simulink model "bh_velocity_estimator"  (R2021a)
settings: Solver=ode15s  StartTime=0.0  StopTime=20  RelTol=1e-3
settings Model: Creator=bhorton  LastModifiedBy=bhorton

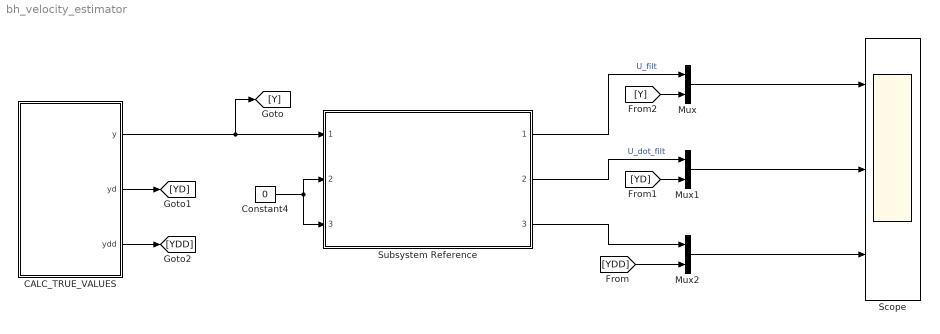
== system bh_velocity_estimator ==
  CALC_TRUE_VALUES : Subsystem
  Constant4 : Constant  Value=0
  Mux : Mux  Inputs=2
  Mux1 : Mux  Inputs=2
  Mux2 : Mux  Inputs=2
  Scope : Scope  NumInputPorts=3
  Subsystem Reference : Subsystem  ReferencedSubsystem=bh_COMPONENT_deriv_est  wn=2*pi*5000  p=1
  wires:
  CALC_TRUE_VALUES/1(y) -> [Y], Subsystem Reference/1
  Constant4/1 -> Subsystem Reference/3, Subsystem Reference/2
  Mux/1 -> Scope/1
  Mux1/1 -> Scope/2
  Mux2/1 -> Scope/3
  Subsystem Reference/1 -> Mux/1  "U_filt"
  Subsystem Reference/2 -> Mux1/1  "U_dot_filt"
  Subsystem Reference/3 -> Mux2/1
  CALC_TRUE_VALUES/3(ydd) -> [YDD]
  CALC_TRUE_VALUES/2(yd) -> [YD]
  [YDD] -> Mux2/2
  [YD] -> Mux1/2
  [Y] -> Mux/2

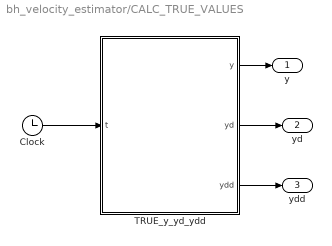
== system bh_velocity_estimator/CALC_TRUE_VALUES ==
  Clock : Clock
  TRUE_y_yd_ydd : MATLAB Function  TreatAsAtomicUnit=on
  y : Outport
  yd : Outport  Port=2
  ydd : Outport  Port=3
  wires:
  TRUE_y_yd_ydd/1(y) -> y/1
  TRUE_y_yd_ydd/3(ydd) -> ydd/1
  TRUE_y_yd_ydd/2(yd) -> yd/1
  Clock/1 -> TRUE_y_yd_ydd/1(t)

== matlab function bh_velocity_estimator/CALC_TRUE_VALUES/TRUE_y_yd_ydd ==
  data: t input; y output; yd output; ydd output
function [y,yd,ydd] = TRUE_y_yd_ydd(t)
%#codegen

%    This function was generated by the Symbolic Math Toolbox version 8.7.
%    11-Aug-2021 12:19:19

t2 = t./5.0;
t3 = sqrt(1.1e+1);
t4 = -t2;
t6 = t.*t3.*(3.0./5.0);
t5 = exp(t4);
t7 = cos(t6);
t8 = sin(t6);
y = t5.*t8.*3.0+t.^2./2.0e+2;
if nargout > 1
    yd = t./1.0e+2-t5.*t8.*(3.0./5.0)+t3.*t5.*t7.*(9.0./5.0);
end
if nargout > 2
    ydd = t5.*t8.*(-2.94e+2./2.5e+1)-t3.*t5.*t7.*(1.8e+1./2.5e+1)+1.0./1.0e+2;
end
